simulink model "chap03_25"  (R2021a)
settings: Solver=FixedStepDiscrete  StartTime=0.0  StopTime=7.5  FixedStep=0.001  RelTol=1e-3
undefined symbols (not defined in the file): DiscIntNeverNeededParam
(part 1 of 2)
settings Model: Creator=陈天兴  LastModifiedBy=陈天兴

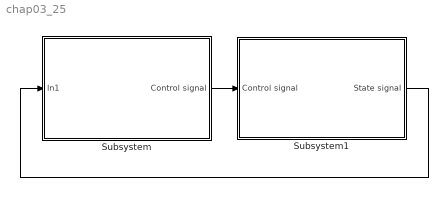
== system chap03_25 ==
  Subsystem : Subsystem
  Subsystem1 : Subsystem
  wires:
  Subsystem1/1(State signal) -> Subsystem/1(In1)
  Subsystem/1(Control signal) -> Subsystem1/1(Control signal)

== system chap03_25/Subsystem ==
  In1 : Inport
  Bus Creator : BusCreator  Inputs=6
  Bus Creator2 : BusCreator  Inputs=1
  Subsystem : Subsystem
  Subsystem1 : Subsystem
  Subsystem2 : Subsystem
  Subsystem3 : Subsystem
  Subsystem4 : Subsystem
  Subsystem5 : Subsystem
  Control signal : Outport
  wires:
  Bus Creator2/1 -> Subsystem4/1(In19), Subsystem1/1(In19), Subsystem3/1(In19), Subsystem/1(In19), Subsystem2/1(In19), Subsystem5/1(In19)
  Subsystem5/1(u3) -> Bus Creator/3
  Subsystem3/1(u4) -> Bus Creator/4
  Subsystem1/1(u5) -> Bus Creator/5
  Subsystem/1(u1) -> Bus Creator/1
  Subsystem2/1(u2) -> Bus Creator/2
  Subsystem4/1(u6) -> Bus Creator/6
  Bus Creator/1 -> Control signal/1
  In1/1 -> Bus Creator2/1  "state(t)"

== system chap03_25/Subsystem1 ==
  Control signal : Inport
  Bus Creator : BusCreator  Inputs=6
  Bus Selector : BusSelector  OutputSignals=node1.ux,node1.uy,node1.uz
  Bus Selector1 : BusSelector  OutputSignals=node2.ux,node2.uy,node2.uz
  Bus Selector2 : BusSelector  OutputSignals=node3.ux,node3.uy,node3.uz
  Bus Selector3 : BusSelector  OutputSignals=node4.ux,node4.uy,node4.uz
  Bus Selector4 : BusSelector  OutputSignals=node5.ux,node5.uy,node5.uz
  Bus Selector5 : BusSelector  OutputSignals=node6.ux,node6.uy,node6.uz
  Subsystem : Subsystem
  Subsystem1 : Subsystem
  Subsystem2 : Subsystem
  Subsystem3 : Subsystem
  Subsystem4 : Subsystem
  Subsystem5 : Subsystem
  State signal : Outport
  wires:
  Bus Creator/1 -> State signal/1
  Subsystem/1(node1) -> Bus Creator/1
  Subsystem1/1(node2) -> Bus Creator/2
  Subsystem2/1(node3) -> Bus Creator/3
  Subsystem3/1(node4) -> Bus Creator/4
  Subsystem4/1(node5) -> Bus Creator/5
  Subsystem5/1(node6) -> Bus Creator/6
  Control signal/1 -> Bus Selector2/1, Bus Selector1/1, Bus Selector/1, Bus Selector5/1, Bus Selector4/1, Bus Selector3/1
  Bus Selector/1 -> Subsystem/1(ut1x)  "<ux>"
  Bus Selector/2 -> Subsystem/2(ut1y)  "<uy>"
  Bus Selector/3 -> Subsystem/3(ut1z)  "<uz>"
  Bus Selector1/1 -> Subsystem1/1(ut2x)  "<ux>"
  Bus Selector1/2 -> Subsystem1/2(ut2y)  "<uy>"
  Bus Selector1/3 -> Subsystem1/3(ut2z)  "<uz>"
  Bus Selector2/1 -> Subsystem2/1(ut3x)  "<ux>"
  Bus Selector2/2 -> Subsystem2/2(ut3y)  "<uy>"
  Bus Selector2/3 -> Subsystem2/3(ut3z)  "<uz>"
  Bus Selector3/1 -> Subsystem3/1(ut4x)  "<ux>"
  Bus Selector3/2 -> Subsystem3/2(ut4y)  "<uy>"
  Bus Selector3/3 -> Subsystem3/3(ut4z)  "<uz>"
  Bus Selector4/1 -> Subsystem4/1(ut5x)  "<ux>"
  Bus Selector4/2 -> Subsystem4/2(ut5y)  "<uy>"
  Bus Selector4/3 -> Subsystem4/3(ut5z)  "<uz>"
  Bus Selector5/1 -> Subsystem5/1(ut6x)  "<ux>"
  Bus Selector5/2 -> Subsystem5/2(ut6y)  "<uy>"
  Bus Selector5/3 -> Subsystem5/3(ut6z)  "<uz>"

== system chap03_25/Subsystem/Subsystem ==
  In19 : Inport
  Bus Creator : BusCreator  Inputs=3
  Bus Selector : BusSelector  OutputSignals=state(t).node1.xx,state(t).node2.xx,state(t).node3.xx,state(t).node6.xx,state(t).node1.vx,state(t).node2.vx,state(t).node3.vx,state(t).node6.vx
  Bus Selector1 : BusSelector  OutputSignals=state(t).node1.xy,state(t).node2.xy,state(t).node3.xy,state(t).node6.xy,state(t).node1.vy,state(t).node2.vy,state(t).node3.vy,state(t).node6.vy
  Bus Selector2 : BusSelector  OutputSignals=state(t).node1.xz,state(t).node2.xz,state(t).node3.xz,state(t).node6.xz,state(t).node1.vz,state(t).node2.vz,state(t).node3.vz,state(t).node6.vz
  Subsystem1 : Subsystem
  Subsystem2 : Subsystem
  Subsystem6 : Subsystem
  u1 : Outport
  wires:
  Subsystem2/1(utx) -> Bus Creator/3  "uz"
  Subsystem6/1(utx) -> Bus Creator/1  "ux"
  Subsystem1/1(utx) -> Bus Creator/2  "uy"
  Bus Creator/1 -> u1/1  "node1"
  In19/1 -> Bus Selector2/1, Bus Selector1/1, Bus Selector/1
  Bus Selector/1 -> Subsystem6/1(xx1)  "<xx>"
  Bus Selector/2 -> Subsystem6/2(xx2)  "<xx>"
  Bus Selector/3 -> Subsystem6/3(xx3)  "<xx>"
  Bus Selector/4 -> Subsystem6/4(xx6)  "<xx>"
  Bus Selector/5 -> Subsystem6/5(vx1)  "<vx>"
  Bus Selector/6 -> Subsystem6/6(vx2)  "<vx>"
  Bus Selector/7 -> Subsystem6/7(vx3)  "<vx>"
  Bus Selector/8 -> Subsystem6/8(vx6)  "<vx>"
  Bus Selector1/1 -> Subsystem1/1(xy1)  "<xy>"
  Bus Selector1/2 -> Subsystem1/2(xy2)  "<xy>"
  Bus Selector1/3 -> Subsystem1/3(xy3)  "<xy>"
  Bus Selector1/4 -> Subsystem1/4(xy6)  "<xy>"
  Bus Selector1/5 -> Subsystem1/5(vy1)  "<vy>"
  Bus Selector1/6 -> Subsystem1/6(vy2)  "<vy>"
  Bus Selector1/7 -> Subsystem1/7(vy3)  "<vy>"
  Bus Selector1/8 -> Subsystem1/8(vy6)  "<vy>"
  Bus Selector2/1 -> Subsystem2/1(xz1)  "<xz>"
  Bus Selector2/2 -> Subsystem2/2(xx2)  "<xz>"
  Bus Selector2/3 -> Subsystem2/3(xz3)  "<xz>"
  Bus Selector2/4 -> Subsystem2/4(xz6)  "<xz>"
  Bus Selector2/5 -> Subsystem2/5(vz1)  "<vz>"
  Bus Selector2/6 -> Subsystem2/6(vz2)  "<vz>"
  Bus Selector2/7 -> Subsystem2/7(vz3)  "<vz>"
  Bus Selector2/8 -> Subsystem2/8(vz6)  "<vz>"

== system chap03_25/Subsystem/Subsystem1 ==
  In19 : Inport
  Bus Creator : BusCreator  Inputs=3
  Bus Selector : BusSelector  OutputSignals=state(t).node5.xx,state(t).node3.xx,state(t).node4.xx,state(t).node5.vx,state(t).node3.vx,state(t).node4.vx
  Bus Selector1 : BusSelector  OutputSignals=state(t).node5.xy,state(t).node3.xy,state(t).node4.xy,state(t).node5.vy,state(t).node3.vy,state(t).node4.vy
  Bus Selector2 : BusSelector  OutputSignals=state(t).node5.xz,state(t).node3.xz,state(t).node4.xz,state(t).node5.vz,state(t).node3.vz,state(t).node4.vz
  Subsystem2 : Subsystem
  Subsystem5 : Subsystem
  Subsystem6 : Subsystem
  u5 : Outport
  wires:
  Bus Creator/1 -> u5/1  "node5"
  Subsystem5/1(uty) -> Bus Creator/2  "uy"
  Subsystem6/1(utx) -> Bus Creator/1  "ux"
  Subsystem2/1(utz) -> Bus Creator/3  "uz"
  Bus Selector1/3 -> Subsystem5/3(xy4)  "<xy>"
  Bus Selector1/2 -> Subsystem5/2(xy3)  "<xy>"
  Bus Selector1/1 -> Subsystem5/1(xy5)  "<xy>"
  Bus Selector2/2 -> Subsystem2/2(xz3)  "<xz>"
  Bus Selector2/6 -> Subsystem2/6(vz4)  "<vz>"
  Bus Selector2/5 -> Subsystem2/5(vz3)  "<vz>"
  Bus Selector/4 -> Subsystem6/4(vx5)  "<vx>"
  Bus Selector1/6 -> Subsystem5/6(vy4)  "<vy>"
  Bus Selector1/4 -> Subsystem5/4(vy5)  "<vy>"
  In19/1 -> Bus Selector2/1, Bus Selector1/1, Bus Selector/1
  Bus Selector/1 -> Subsystem6/1(xx5)  "<xx>"
  Bus Selector/2 -> Subsystem6/2(xx3)  "<xx>"
  Bus Selector1/5 -> Subsystem5/5(vy3)  "<vy>"
  Bus Selector/6 -> Subsystem6/6(vx4)  "<vx>"
  Bus Selector/5 -> Subsystem6/5(vx3)  "<vx>"
  Bus Selector/3 -> Subsystem6/3(xx4)  "<xx>"
  Bus Selector2/1 -> Subsystem2/1(xz5)  "<xz>"
  Bus Selector2/3 -> Subsystem2/3(xz4)  "<xz>"
  Bus Selector2/4 -> Subsystem2/4(vz5)  "<vz>"

== system chap03_25/Subsystem/Subsystem2 ==
  In19 : Inport
  Bus Creator : BusCreator  Inputs=3
  Bus Selector : BusSelector  OutputSignals=state(t).node2.xx,state(t).node1.xx,state(t).node4.xx,state(t).node6.xx,state(t).node2.vx,state(t).node1.vx,state(t).node4.vx,state(t).node6.vx
  Bus Selector1 : BusSelector  OutputSignals=state(t).node2.xy,state(t).node1.xy,state(t).node4.xy,state(t).node6.xy,state(t).node2.vy,state(t).node1.vy,state(t).node4.vy,state(t).node6.vy
  Bus Selector2 : BusSelector  OutputSignals=state(t).node2.xz,state(t).node1.xz,state(t).node4.xz,state(t).node6.xz,state(t).node2.vz,state(t).node1.vz,state(t).node4.vz,state(t).node6.vz
  Subsystem1 : Subsystem
  Subsystem2 : Subsystem
  Subsystem6 : Subsystem
  u2 : Outport
  wires:
  Bus Creator/1 -> u2/1  "node2"
  Subsystem1/1(uty) -> Bus Creator/2  "uy"
  Subsystem6/1(utx) -> Bus Creator/1  "ux"
  Subsystem2/1(utz) -> Bus Creator/3  "uz"
  Bus Selector2/1 -> Subsystem2/1(xz2)  "<xz>"
  In19/1 -> Bus Selector2/1, Bus Selector1/1, Bus Selector/1
  Bus Selector/3 -> Subsystem6/3(xx4)  "<xx>"
  Bus Selector/5 -> Subsystem6/5(vx2)  "<vx>"
  Bus Selector/1 -> Subsystem6/1(xx2)  "<xx>"
  Bus Selector/7 -> Subsystem6/7(vx4)  "<vx>"
  Bus Selector1/2 -> Subsystem1/2(xy1)  "<xy>"
  Bus Selector2/4 -> Subsystem2/4(xz6)  "<xz>"
  Bus Selector2/6 -> Subsystem2/6(vz1)  "<vz>"
  Bus Selector1/1 -> Subsystem1/1(xy2)  "<xy>"
  Bus Selector2/7 -> Subsystem2/7(vz4)  "<vz>"
  Bus Selector2/5 -> Subsystem2/5(vz2)  "<vz>"
  Bus Selector1/6 -> Subsystem1/6(vy1)  "<vy>"
  Bus Selector/2 -> Subsystem6/2(xx1)  "<xx>"
  Bus Selector1/8 -> Subsystem1/8(vy6)  "<vy>"
  Bus Selector2/8 -> Subsystem2/8(vz6)  "<vz>"
  Bus Selector1/7 -> Subsystem1/7(vy4)  "<vy>"
  Bus Selector2/2 -> Subsystem2/2(xz1)  "<xz>"
  Bus Selector/8 -> Subsystem6/8(vx6)  "<vx>"
  Bus Selector1/3 -> Subsystem1/3(xy4)  "<xy>"
  Bus Selector/6 -> Subsystem6/6(vx1)  "<vx>"
  Bus Selector1/4 -> Subsystem1/4(xy6)  "<xy>"
  Bus Selector1/5 -> Subsystem1/5(vy2)  "<vy>"
  Bus Selector2/3 -> Subsystem2/3(xz4)  "<xz>"
  Bus Selector/4 -> Subsystem6/4(xx6)  "<xx>"

== system chap03_25/Subsystem/Subsystem3 ==
  In19 : Inport
  Bus Creator : BusCreator  Inputs=3
  Bus Selector : BusSelector  OutputSignals=state(t).node4.xx,state(t).node2.xx,state(t).node3.xx,state(t).node5.xx,state(t).node4.vx,state(t).node2.vx,state(t).node3.vx,state(t).node5.vx
  Bus Selector1 : BusSelector  OutputSignals=state(t).node4.xy,state(t).node2.xy,state(t).node3.xy,state(t).node5.xy,state(t).node4.vy,state(t).node2.vy,state(t).node3.vy,state(t).node5.vy
  Bus Selector2 : BusSelector  OutputSignals=state(t).node4.xz,state(t).node2.xz,state(t).node3.xz,state(t).node5.xz,state(t).node4.vz,state(t).node2.vz,state(t).node3.vz,state(t).node5.vz
  Subsystem1 : Subsystem
  Subsystem2 : Subsystem
  Subsystem6 : Subsystem
  u4 : Outport
  wires:
  Bus Creator/1 -> u4/1  "node4"
  Subsystem1/1(utx) -> Bus Creator/2  "uy"
  Subsystem6/1(utx) -> Bus Creator/1  "ux"
  Subsystem2/1(utx) -> Bus Creator/3  "uz"
  Bus Selector/2 -> Subsystem6/2(xx2)  "<xx>"
  Bus Selector1/7 -> Subsystem1/7(vy3)  "<vy>"
  Bus Selector1/4 -> Subsystem1/4(xy5)  "<xy>"
  Bus Selector2/3 -> Subsystem2/3(xz3)  "<xz>"
  Bus Selector/8 -> Subsystem6/8(vx5)  "<vx>"
  Bus Selector2/2 -> Subsystem2/2(xx2)  "<xz>"
  Bus Selector2/4 -> Subsystem2/4(xz5)  "<xz>"
  Bus Selector1/5 -> Subsystem1/5(vy4)  "<vy>"
  Bus Selector1/2 -> Subsystem1/2(xy2)  "<xy>"
  Bus Selector2/7 -> Subsystem2/7(vz3)  "<vz>"
  Bus Selector2/5 -> Subsystem2/5(vz4)  "<vz>"
  Bus Selector1/6 -> Subsystem1/6(vy2)  "<vy>"
  Bus Selector2/8 -> Subsystem2/8(vz5)  "<vz>"
  Bus Selector2/6 -> Subsystem2/6(vz2)  "<vz>"
  Bus Selector1/3 -> Subsystem1/3(xy3)  "<xy>"
  Bus Selector2/1 -> Subsystem2/1(xz4)  "<xz>"
  Bus Selector/5 -> Subsystem6/5(vx4)  "<vx>"
  Bus Selector/1 -> Subsystem6/1(xx4)  "<xx>"
  Bus Selector/3 -> Subsystem6/3(xx3)  "<xx>"
  In19/1 -> Bus Selector2/1, Bus Selector1/1, Bus Selector/1
  Bus Selector1/8 -> Subsystem1/8(vy5)  "<vy>"
  Bus Selector1/1 -> Subsystem1/1(xy4)  "<xy>"
  Bus Selector/7 -> Subsystem6/7(vx3)  "<vx>"
  Bus Selector/6 -> Subsystem6/6(vx2)  "<vx>"
  Bus Selector/4 -> Subsystem6/4(xx5)  "<xx>"

== system chap03_25/Subsystem/Subsystem4 ==
  In19 : Inport
  Bus Creator : BusCreator  Inputs=3
  Bus Selector : BusSelector  OutputSignals=state(t).node6.xx,state(t).node1.xx,state(t).node2.xx,state(t).node6.vx,state(t).node1.vx,state(t).node2.vx
  Bus Selector1 : BusSelector  OutputSignals=state(t).node6.xy,state(t).node1.xy,state(t).node2.xy,state(t).node6.vy,state(t).node1.vy,state(t).node2.vy
  Bus Selector2 : BusSelector  OutputSignals=state(t).node6.xz,state(t).node1.xz,state(t).node2.xz,state(t).node6.vz,state(t).node1.vz,state(t).node2.vz
  Subsystem1 : Subsystem
  Subsystem2 : Subsystem
  Subsystem6 : Subsystem
  u6 : Outport
  wires:
  Subsystem2/1(utz) -> Bus Creator/3  "uz"
  Subsystem6/1(utx) -> Bus Creator/1  "ux"
  Subsystem1/1(uty) -> Bus Creator/2  "uy"
  Bus Creator/1 -> u6/1  "node6"
  Bus Selector/1 -> Subsystem6/1(xx6)  "<xx>"
  Bus Selector/2 -> Subsystem6/2(xx1)  "<xx>"
  In19/1 -> Bus Selector2/1, Bus Selector1/1, Bus Selector/1
  Bus Selector2/3 -> Subsystem2/3(xz2)  "<xz>"
  Bus Selector/3 -> Subsystem6/3(xx2)  "<xx>"
  Bus Selector1/1 -> Subsystem1/1(xy6)  "<xy>"
  Bus Selector/4 -> Subsystem6/4(vx6)  "<vx>"
  Bus Selector1/2 -> Subsystem1/2(xy1)  "<xy>"
  Bus Selector/5 -> Subsystem6/5(vx1)  "<vx>"
  Bus Selector1/3 -> Subsystem1/3(xy2)  "<xy>"
  Bus Selector2/5 -> Subsystem2/5(vz1)  "<vz>"
  Bus Selector1/4 -> Subsystem1/4(vy6)  "<vy>"
  Bus Selector1/5 -> Subsystem1/5(vy1)  "<vy>"
  Bus Selector1/6 -> Subsystem1/6(vy2)  "<vy>"
  Bus Selector2/4 -> Subsystem2/4(vz6)  "<vz>"
  Bus Selector/6 -> Subsystem6/6(vx2)  "<vx>"
  Bus Selector2/2 -> Subsystem2/2(xz1)  "<xz>"
  Bus Selector2/1 -> Subsystem2/1(xz6)  "<xz>"
  Bus Selector2/6 -> Subsystem2/6(vz2)  "<vz>"

== system chap03_25/Subsystem/Subsystem5 ==
  In19 : Inport
  Bus Creator : BusCreator  Inputs=3
  Bus Selector : BusSelector  OutputSignals=state(t).node3.xx,state(t).node1.xx,state(t).node4.xx,state(t).node5.xx,state(t).node3.vx,state(t).node1.vx,state(t).node4.vx,state(t).node5.vx
  Bus Selector1 : BusSelector  OutputSignals=state(t).node3.xy,state(t).node1.xy,state(t).node4.xy,state(t).node5.xy,state(t).node3.vy,state(t).node1.vy,state(t).node4.vy,state(t).node5.vy
  Bus Selector2 : BusSelector  OutputSignals=state(t).node3.xz,state(t).node1.xz,state(t).node4.xz,state(t).node5.xz,state(t).node3.vz,state(t).node1.vz,state(t).node4.vz,state(t).node5.vz
  Subsystem1 : Subsystem
  Subsystem2 : Subsystem
  Subsystem6 : Subsystem
  u3 : Outport
  wires:
  Subsystem2/1(utz) -> Bus Creator/3  "uz"
  Subsystem6/1(utx) -> Bus Creator/1  "ux"
  Subsystem1/1(uty) -> Bus Creator/2  "uy"
  Bus Creator/1 -> u3/1  "node3"
  Bus Selector/7 -> Subsystem6/7(vx4)  "<vx>"
  In19/1 -> Bus Selector2/1, Bus Selector1/1, Bus Selector/1
  Bus Selector2/6 -> Subsystem2/6(vz1)  "<vz>"
  Bus Selector/8 -> Subsystem6/8(vx5)  "<vx>"
  Bus Selector1/1 -> Subsystem1/1(xy3)  "<xy>"
  Bus Selector/2 -> Subsystem6/2(xx1)  "<xx>"
  Bus Selector2/3 -> Subsystem2/3(xz4)  "<xz>"
  Bus Selector2/2 -> Subsystem2/2(xz1)  "<xz>"
  Bus Selector/5 -> Subsystem6/5(vx3)  "<vx>"
  Bus Selector/1 -> Subsystem6/1(xx3)  "<xx>"
  Bus Selector1/7 -> Subsystem1/7(vy4)  "<vy>"
  Bus Selector/3 -> Subsystem6/3(xx4)  "<xx>"
  Bus Selector/6 -> Subsystem6/6(vx1)  "<vx>"
  Bus Selector1/2 -> Subsystem1/2(xy1)  "<xy>"
  Bus Selector1/5 -> Subsystem1/5(vy3)  "<vy>"
  Bus Selector1/8 -> Subsystem1/8(vy5)  "<vy>"
  Bus Selector2/1 -> Subsystem2/1(xz3)  "<xz>"
  Bus Selector1/4 -> Subsystem1/4(xy5)  "<xy>"
  Bus Selector1/3 -> Subsystem1/3(xy4)  "<xy>"
  Bus Selector/4 -> Subsystem6/4(xx5)  "<xx>"
  Bus Selector2/5 -> Subsystem2/5(vz3)  "<vz>"
  Bus Selector2/7 -> Subsystem2/7(vz4)  "<vz>"
  Bus Selector1/6 -> Subsystem1/6(vy1)  "<vy>"
  Bus Selector2/8 -> Subsystem2/8(vz5)  "<vz>"
  Bus Selector2/4 -> Subsystem2/4(xz5)  "<xz>"

== system chap03_25/Subsystem1/Subsystem ==
  ut1x : Inport
  ut1y : Inport  Port=2
  ut1z : Inport  Port=3
  Bus Creator1 : BusCreator  Inputs=6
  Discrete-Time Integrator : DiscreteIntegrator  SampleTime=-1  ICPrevOutput=DiscIntNeverNeededParam  ICPrevScaledInput=DiscIntNeverNeededParam
  Discrete-Time Integrator14 : DiscreteIntegrator  InitialCondition=-2.7  SampleTime=-1  ICPrevOutput=DiscIntNeverNeededParam  ICPrevScaledInput=DiscIntNeverNeededParam
  Discrete-Time Integrator15 : DiscreteIntegrator  InitialCondition=2.5  SampleTime=-1  ICPrevOutput=DiscIntNeverNeededParam  ICPrevScaledInput=DiscIntNeverNeededParam
  Discrete-Time Integrator16 : DiscreteIntegrator  InitialCondition=0.17  SampleTime=-1  ICPrevOutput=DiscIntNeverNeededParam  ICPrevScaledInput=DiscIntNeverNeededParam
  Discrete-Time Integrator17 : DiscreteIntegrator  SampleTime=-1  ICPrevOutput=DiscIntNeverNeededParam  ICPrevScaledInput=DiscIntNeverNeededParam
  Discrete-Time Integrator5 : DiscreteIntegrator  InitialCondition=-2.9  SampleTime=-1  ICPrevOutput=DiscIntNeverNeededParam  ICPrevScaledInput=DiscIntNeverNeededParam
  node1 : Outport
  wires:
  ut1y/1 -> Discrete-Time Integrator17/1
  ut1z/1 -> Discrete-Time Integrator/1
  Discrete-Time Integrator17/1 -> Discrete-Time Integrator15/1, Bus Creator1/5  "vy"
  Discrete-Time Integrator/1 -> Discrete-Time Integrator5/1, Bus Creator1/6  "vz"
  ut1x/1 -> Discrete-Time Integrator16/1
  Discrete-Time Integrator16/1 -> Bus Creator1/4, Discrete-Time Integrator14/1  "vx"
  Bus Creator1/1 -> node1/1  "node1"
  Discrete-Time Integrator5/1 -> Bus Creator1/3  "xz"
  Discrete-Time Integrator15/1 -> Bus Creator1/2  "xy"
  Discrete-Time Integrator14/1 -> Bus Creator1/1  "xx"

== system chap03_25/Subsystem1/Subsystem1 ==
  ut2x : Inport
  ut2y : Inport  Port=2
  ut2z : Inport  Port=3
  Bus Creator1 : BusCreator  Inputs=6
  Discrete-Time Integrator1 : DiscreteIntegrator  SampleTime=-1  ICPrevOutput=DiscIntNeverNeededParam  ICPrevScaledInput=DiscIntNeverNeededParam
  Discrete-Time Integrator14 : DiscreteIntegrator  InitialCondition=-1.7  SampleTime=-1  ICPrevOutput=DiscIntNeverNeededParam  ICPrevScaledInput=DiscIntNeverNeededParam
  Discrete-Time Integrator15 : DiscreteIntegrator  InitialCondition=-1.4  SampleTime=-1  ICPrevOutput=DiscIntNeverNeededParam  ICPrevScaledInput=DiscIntNeverNeededParam
  Discrete-Time Integrator2 : DiscreteIntegrator  SampleTime=-1  ICPrevOutput=DiscIntNeverNeededParam  ICPrevScaledInput=DiscIntNeverNeededParam
  Discrete-Time Integrator3 : DiscreteIntegrator  InitialCondition=0.13  SampleTime=-1  ICPrevOutput=DiscIntNeverNeededParam  ICPrevScaledInput=DiscIntNeverNeededParam
  Discrete-Time Integrator5 : DiscreteIntegrator  InitialCondition=-1.5  SampleTime=-1  ICPrevOutput=DiscIntNeverNeededParam  ICPrevScaledInput=DiscIntNeverNeededParam
  node2 : Outport
  wires:
  Discrete-Time Integrator14/1 -> Bus Creator1/1  "xx"
  Discrete-Time Integrator15/1 -> Bus Creator1/2  "xy"
  Discrete-Time Integrator5/1 -> Bus Creator1/3  "xz"
  Bus Creator1/1 -> node2/1  "node2"
  Discrete-Time Integrator2/1 -> Discrete-Time Integrator14/1, Bus Creator1/4  "vx"
  ut2x/1 -> Discrete-Time Integrator2/1
  Discrete-Time Integrator1/1 -> Bus Creator1/6, Discrete-Time Integrator5/1  "vz"
  Discrete-Time Integrator3/1 -> Bus Creator1/5, Discrete-Time Integrator15/1  "vy"
  ut2z/1 -> Discrete-Time Integrator1/1
  ut2y/1 -> Discrete-Time Integrator3/1

== system chap03_25/Subsystem1/Subsystem2 ==
  ut3x : Inport
  ut3y : Inport  Port=2
  ut3z : Inport  Port=3
  Bus Creator1 : BusCreator  Inputs=6
  Discrete-Time Integrator : DiscreteIntegrator  InitialCondition=0.12  SampleTime=-1  ICPrevOutput=DiscIntNeverNeededParam  ICPrevScaledInput=DiscIntNeverNeededParam
  Discrete-Time Integrator14 : DiscreteIntegrator  InitialCondition=0.6  SampleTime=-1  ICPrevOutput=DiscIntNeverNeededParam  ICPrevScaledInput=DiscIntNeverNeededParam
  Discrete-Time Integrator15 : DiscreteIntegrator  InitialCondition=-0.7  SampleTime=-1  ICPrevOutput=DiscIntNeverNeededParam  ICPrevScaledInput=DiscIntNeverNeededParam
  Discrete-Time Integrator16 : DiscreteIntegrator  SampleTime=-1  ICPrevOutput=DiscIntNeverNeededParam  ICPrevScaledInput=DiscIntNeverNeededParam
  Discrete-Time Integrator17 : DiscreteIntegrator  SampleTime=-1  ICPrevOutput=DiscIntNeverNeededParam  ICPrevScaledInput=DiscIntNeverNeededParam
  Discrete-Time Integrator5 : DiscreteIntegrator  InitialCondition=0.5  SampleTime=-1  ICPrevOutput=DiscIntNeverNeededParam  ICPrevScaledInput=DiscIntNeverNeededParam
  node3 : Outport
  wires:
  ut3y/1 -> Discrete-Time Integrator17/1
  ut3z/1 -> Discrete-Time Integrator/1
  Discrete-Time Integrator17/1 -> Discrete-Time Integrator15/1, Bus Creator1/5  "vy"
  Discrete-Time Integrator/1 -> Discrete-Time Integrator5/1, Bus Creator1/6  "vz"
  ut3x/1 -> Discrete-Time Integrator16/1
  Discrete-Time Integrator16/1 -> Bus Creator1/4, Discrete-Time Integrator14/1  "vx"
  Bus Creator1/1 -> node3/1  "node3"
  Discrete-Time Integrator5/1 -> Bus Creator1/3  "xz"
  Discrete-Time Integrator15/1 -> Bus Creator1/2  "xy"
  Discrete-Time Integrator14/1 -> Bus Creator1/1  "xx"

== system chap03_25/Subsystem1/Subsystem3 ==
  ut4x : Inport
  ut4y : Inport  Port=2
  ut4z : Inport  Port=3
  Bus Creator1 : BusCreator  Inputs=6
  Discrete-Time Integrator : DiscreteIntegrator  InitialCondition=-0.15  SampleTime=-1  ICPrevOutput=DiscIntNeverNeededParam  ICPrevScaledInput=DiscIntNeverNeededParam
  Discrete-Time Integrator14 : DiscreteIntegrator  InitialCondition=-0.7  SampleTime=-1  ICPrevOutput=DiscIntNeverNeededParam  ICPrevScaledInput=DiscIntNeverNeededParam
  Discrete-Time Integrator15 : DiscreteIntegrator  InitialCondition=0.9  SampleTime=-1  ICPrevOutput=DiscIntNeverNeededParam  ICPrevScaledInput=DiscIntNeverNeededParam
  Discrete-Time Integrator16 : DiscreteIntegrator  SampleTime=-1  ICPrevOutput=DiscIntNeverNeededParam  ICPrevScaledInput=DiscIntNeverNeededParam
  Discrete-Time Integrator17 : DiscreteIntegrator  SampleTime=-1  ICPrevOutput=DiscIntNeverNeededParam  ICPrevScaledInput=DiscIntNeverNeededParam
  Discrete-Time Integrator5 : DiscreteIntegrator  InitialCondition=-0.8  SampleTime=-1  ICPrevOutput=DiscIntNeverNeededParam  ICPrevScaledInput=DiscIntNeverNeededParam
  node4 : Outport
  wires:
  Discrete-Time Integrator14/1 -> Bus Creator1/1  "xx"
  Discrete-Time Integrator15/1 -> Bus Creator1/2  "xy"
  Discrete-Time Integrator5/1 -> Bus Creator1/3  "xz"
  Bus Creator1/1 -> node4/1  "node4"
  Discrete-Time Integrator16/1 -> Discrete-Time Integrator14/1, Bus Creator1/4  "vx"
  ut4x/1 -> Discrete-Time Integrator16/1
  Discrete-Time Integrator/1 -> Bus Creator1/6, Discrete-Time Integrator5/1  "vz"
  Discrete-Time Integrator17/1 -> Bus Creator1/5, Discrete-Time Integrator15/1  "vy"
  ut4z/1 -> Discrete-Time Integrator/1
  ut4y/1 -> Discrete-Time Integrator17/1

== system chap03_25/Subsystem1/Subsystem4 ==
  ut5x : Inport
  ut5y : Inport  Port=2
  ut5z : Inport  Port=3
  Bus Creator1 : BusCreator  Inputs=6
  Discrete-Time Integrator : DiscreteIntegrator  SampleTime=-1  ICPrevOutput=DiscIntNeverNeededParam  ICPrevScaledInput=DiscIntNeverNeededParam
  Discrete-Time Integrator14 : DiscreteIntegrator  InitialCondition=1.1  SampleTime=-1  ICPrevOutput=DiscIntNeverNeededParam  ICPrevScaledInput=DiscIntNeverNeededParam
  Discrete-Time Integrator15 : DiscreteIntegrator  InitialCondition=1.6  SampleTime=-1  ICPrevOutput=DiscIntNeverNeededParam  ICPrevScaledInput=DiscIntNeverNeededParam
  Discrete-Time Integrator16 : DiscreteIntegrator  SampleTime=-1  ICPrevOutput=DiscIntNeverNeededParam  ICPrevScaledInput=DiscIntNeverNeededParam
  Discrete-Time Integrator17 : DiscreteIntegrator  InitialCondition=-0.12  SampleTime=-1  ICPrevOutput=DiscIntNeverNeededParam  ICPrevScaledInput=DiscIntNeverNeededParam
  Discrete-Time Integrator5 : DiscreteIntegrator  InitialCondition=1.4  SampleTime=-1  ICPrevOutput=DiscIntNeverNeededParam  ICPrevScaledInput=DiscIntNeverNeededParam
  node5 : Outport
  wires:
  ut5y/1 -> Discrete-Time Integrator17/1
  ut5z/1 -> Discrete-Time Integrator/1
  Discrete-Time Integrator17/1 -> Discrete-Time Integrator15/1, Bus Creator1/5  "vy"
  Discrete-Time Integrator/1 -> Discrete-Time Integrator5/1, Bus Creator1/6  "vz"
  ut5x/1 -> Discrete-Time Integrator16/1
  Discrete-Time Integrator16/1 -> Bus Creator1/4, Discrete-Time Integrator14/1  "vx"
  Bus Creator1/1 -> node5/1  "node5"
  Discrete-Time Integrator5/1 -> Bus Creator1/3  "xz"
  Discrete-Time Integrator15/1 -> Bus Creator1/2  "xy"
  Discrete-Time Integrator14/1 -> Bus Creator1/1  "xx"

== system chap03_25/Subsystem1/Subsystem5 ==
  ut6x : Inport
  ut6y : Inport  Port=2
  ut6z : Inport  Port=3
  Bus Creator1 : BusCreator  Inputs=6
  Discrete-Time Integrator : DiscreteIntegrator  SampleTime=-1  ICPrevOutput=DiscIntNeverNeededParam  ICPrevScaledInput=DiscIntNeverNeededParam
  Discrete-Time Integrator14 : DiscreteIntegrator  InitialCondition=2.7  SampleTime=-1  ICPrevOutput=DiscIntNeverNeededParam  ICPrevScaledInput=DiscIntNeverNeededParam
  Discrete-Time Integrator15 : DiscreteIntegrator  InitialCondition=-2.8  SampleTime=-1  ICPrevOutput=DiscIntNeverNeededParam  ICPrevScaledInput=DiscIntNeverNeededParam
  Discrete-Time Integrator16 : DiscreteIntegrator  InitialCondition=-0.18  SampleTime=-1  ICPrevOutput=DiscIntNeverNeededParam  ICPrevScaledInput=DiscIntNeverNeededParam
  Discrete-Time Integrator17 : DiscreteIntegrator  SampleTime=-1  ICPrevOutput=DiscIntNeverNeededParam  ICPrevScaledInput=DiscIntNeverNeededParam
  Discrete-Time Integrator5 : DiscreteIntegrator  InitialCondition=2.5  SampleTime=-1  ICPrevOutput=DiscIntNeverNeededParam  ICPrevScaledInput=DiscIntNeverNeededParam
  node6 : Outport
  wires:
  Discrete-Time Integrator14/1 -> Bus Creator1/1  "xx"
  Discrete-Time Integrator15/1 -> Bus Creator1/2  "xy"
  Discrete-Time Integrator5/1 -> Bus Creator1/3  "xz"
  Bus Creator1/1 -> node6/1  "node6"
  Discrete-Time Integrator16/1 -> Discrete-Time Integrator14/1, Bus Creator1/4  "vx"
  ut6x/1 -> Discrete-Time Integrator16/1
  Discrete-Time Integrator/1 -> Bus Creator1/6, Discrete-Time Integrator5/1  "vz"
  Discrete-Time Integrator17/1 -> Bus Creator1/5, Discrete-Time Integrator15/1  "vy"
  ut6z/1 -> Discrete-Time Integrator/1
  ut6y/1 -> Discrete-Time Integrator17/1

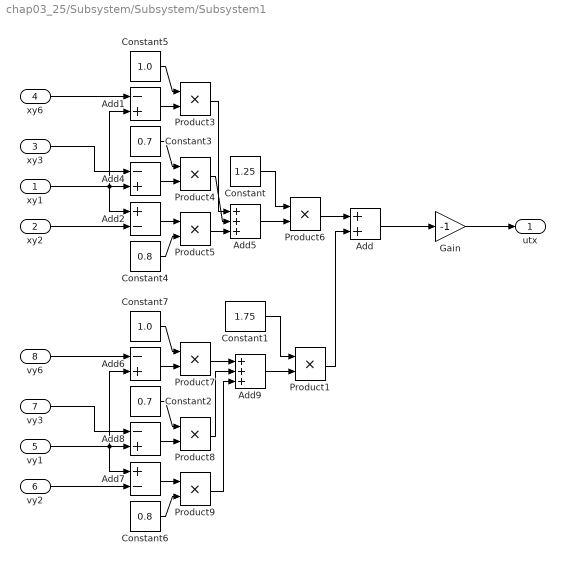
== system chap03_25/Subsystem/Subsystem/Subsystem1 ==
  xy1 : Inport
  xy2 : Inport  Port=2
  xy3 : Inport  Port=3
  xy6 : Inport  Port=4
  vy1 : Inport  Port=5
  vy2 : Inport  Port=6
  vy3 : Inport  Port=7
  vy6 : Inport  Port=8
  Add : Sum
  Add{1,4,6,8} (4 alike) : Sum  Inputs=-+
  Add2 : Sum  Inputs=+-
  Add5 : Sum  Inputs=+++
  Add7 : Sum  Inputs=+-
  Add9 : Sum  Inputs=+++
  Constant : Constant  Value=1.25
  Constant1 : Constant  Value=1.75
  Constant2 : Constant  Value=0.7
  Constant3 : Constant  Value=0.7
  Constant4 : Constant  Value=0.8
  Constant5 : Constant  Value=1.0
  Constant6 : Constant  Value=0.8
  Constant7 : Constant  Value=1.0
  Gain : Gain  Gain=-1
  Product{1,3..9} (8 alike) : Product
  utx : Outport
  wires:
  Product8/1 -> Add9/2
  Product9/1 -> Add9/3
  Constant2/1 -> Product8/1
  Add8/1 -> Product8/2
  vy1/1 -> Add6/2, Add8/2, Add7/1
  Constant6/1 -> Product9/2
  Add7/1 -> Product9/1
  vy3/1 -> Add8/1
  vy2/1 -> Add7/2
  vy6/1 -> Add6/1
  Constant7/1 -> Product7/1
  Add6/1 -> Product7/2
  Product7/1 -> Add9/1
  Product3/1 -> Add5/1
  Add1/1 -> Product3/2
  Constant5/1 -> Product3/1
  xy6/1 -> Add1/1
  xy2/1 -> Add2/2
  xy3/1 -> Add4/1
  Add5/1 -> Product6/2
  Add2/1 -> Product5/1
  Product1/1 -> Add/2
  Constant1/1 -> Product1/1
  Constant/1 -> Product6/1
  Product6/1 -> Add/1
  Constant4/1 -> Product5/2
  xy1/1 -> Add2/1, Add4/2, Add1/2
  Add4/1 -> Product4/2
  Constant3/1 -> Product4/1
  Product5/1 -> Add5/3
  Product4/1 -> Add5/2
  Add9/1 -> Product1/2
  Gain/1 -> utx/1
  Add/1 -> Gain/1

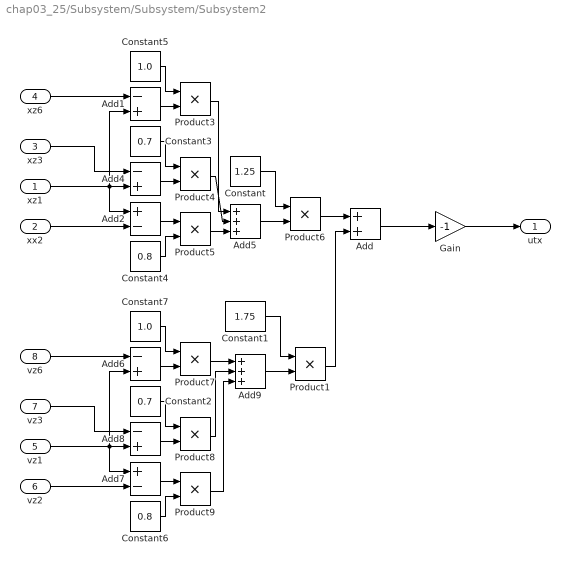
== system chap03_25/Subsystem/Subsystem/Subsystem2 ==
  xz1 : Inport
  xx2 : Inport  Port=2
  xz3 : Inport  Port=3
  xz6 : Inport  Port=4
  vz1 : Inport  Port=5
  vz2 : Inport  Port=6
  vz3 : Inport  Port=7
  vz6 : Inport  Port=8
  Add : Sum
  Add{1,4,6,8} (4 alike) : Sum  Inputs=-+
  Add2 : Sum  Inputs=+-
  Add5 : Sum  Inputs=+++
  Add7 : Sum  Inputs=+-
  Add9 : Sum  Inputs=+++
  Constant : Constant  Value=1.25
  Constant1 : Constant  Value=1.75
  Constant2 : Constant  Value=0.7
  Constant3 : Constant  Value=0.7
  Constant4 : Constant  Value=0.8
  Constant5 : Constant  Value=1.0
  Constant6 : Constant  Value=0.8
  Constant7 : Constant  Value=1.0
  Gain : Gain  Gain=-1
  Product{1,3..9} (8 alike) : Product
  utx : Outport
  wires:
  Add9/1 -> Product1/2
  Product4/1 -> Add5/2
  Product5/1 -> Add5/3
  Constant3/1 -> Product4/1
  Add4/1 -> Product4/2
  xz1/1 -> Add1/2, Add4/2, Add2/1
  Constant4/1 -> Product5/2
  Product6/1 -> Add/1
  Constant/1 -> Product6/1
  Constant1/1 -> Product1/1
  Product1/1 -> Add/2
  Add2/1 -> Product5/1
  Add5/1 -> Product6/2
  xz3/1 -> Add4/1
  xx2/1 -> Add2/2
  xz6/1 -> Add1/1
  Constant5/1 -> Product3/1
  Add1/1 -> Product3/2
  Product3/1 -> Add5/1
  Product7/1 -> Add9/1
  Add6/1 -> Product7/2
  Constant7/1 -> Product7/1
  vz6/1 -> Add6/1
  vz2/1 -> Add7/2
  vz3/1 -> Add8/1
  Add7/1 -> Product9/1
  Constant6/1 -> Product9/2
  vz1/1 -> Add7/1, Add8/2, Add6/2
  Add8/1 -> Product8/2
  Constant2/1 -> Product8/1
  Product9/1 -> Add9/3
  Product8/1 -> Add9/2
  Gain/1 -> utx/1
  Add/1 -> Gain/1

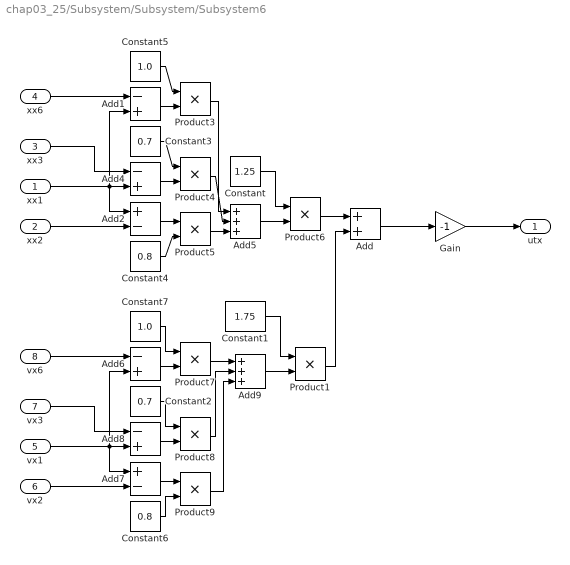
== system chap03_25/Subsystem/Subsystem/Subsystem6 ==
  xx1 : Inport
  xx2 : Inport  Port=2
  xx3 : Inport  Port=3
  xx6 : Inport  Port=4
  vx1 : Inport  Port=5
  vx2 : Inport  Port=6
  vx3 : Inport  Port=7
  vx6 : Inport  Port=8
  Add : Sum
  Add{1,4,6,8} (4 alike) : Sum  Inputs=-+
  Add2 : Sum  Inputs=+-
  Add5 : Sum  Inputs=+++
  Add7 : Sum  Inputs=+-
  Add9 : Sum  Inputs=+++
  Constant : Constant  Value=1.25
  Constant1 : Constant  Value=1.75
  Constant2 : Constant  Value=0.7
  Constant3 : Constant  Value=0.7
  Constant4 : Constant  Value=0.8
  Constant5 : Constant  Value=1.0
  Constant6 : Constant  Value=0.8
  Constant7 : Constant  Value=1.0
  Gain : Gain  Gain=-1
  Product{1,3..9} (8 alike) : Product
  utx : Outport
  wires:
  Add9/1 -> Product1/2
  Product4/1 -> Add5/2
  Product5/1 -> Add5/3
  Constant3/1 -> Product4/1
  Add4/1 -> Product4/2
  xx1/1 -> Add1/2, Add4/2, Add2/1
  Constant4/1 -> Product5/2
  Product6/1 -> Add/1
  Constant/1 -> Product6/1
  Constant1/1 -> Product1/1
  Product1/1 -> Add/2
  Add2/1 -> Product5/1
  Add5/1 -> Product6/2
  Add/1 -> Gain/1
  xx3/1 -> Add4/1
  xx2/1 -> Add2/2
  xx6/1 -> Add1/1
  Constant5/1 -> Product3/1
  Add1/1 -> Product3/2
  Product3/1 -> Add5/1
  Product7/1 -> Add9/1
  Add6/1 -> Product7/2
  Constant7/1 -> Product7/1
  vx6/1 -> Add6/1
  vx2/1 -> Add7/2
  vx3/1 -> Add8/1
  Add7/1 -> Product9/1
  Constant6/1 -> Product9/2
  vx1/1 -> Add7/1, Add8/2, Add6/2
  Add8/1 -> Product8/2
  Constant2/1 -> Product8/1
  Product9/1 -> Add9/3
  Product8/1 -> Add9/2
  Gain/1 -> utx/1

== system chap03_25/Subsystem/Subsystem1/Subsystem2 ==
  xz5 : Inport
  xz3 : Inport  Port=2
  xz4 : Inport  Port=3
  vz5 : Inport  Port=4
  vz3 : Inport  Port=5
  vz4 : Inport  Port=6
  Add : Sum
  Add10 : Sum  Inputs=-+
  Add2 : Sum  Inputs=+-
  Add4 : Sum  Inputs=-+
  Add5 : Sum
  Add8 : Sum
  Add9 : Sum  Inputs=+-
  Constant : Constant  Value=1.25
  Constant1 : Constant  Value=1.75
  Constant3 : Constant  Value=1.0
  Constant4 : Constant  Value=1.2
  Constant5 : Constant  Value=1.0
  Constant6 : Constant  Value=1.2
  Gain : Gain  Gain=-1
  Product{1,4..6,8..9} (6 alike) : Product
  utz : Outport
  wires:
  vz5/1 -> Add9/1, Add10/2
  vz4/1 -> Add10/1
  vz3/1 -> Add9/2
  xz3/1 -> Add2/2
  xz4/1 -> Add4/1
  Add5/1 -> Product6/2
  Add2/1 -> Product5/1
  Product1/1 -> Add/2
  Constant1/1 -> Product1/1
  Constant/1 -> Product6/1
  Product6/1 -> Add/1
  Constant4/1 -> Product5/2
  xz5/1 -> Add4/2, Add2/1
  Add4/1 -> Product4/2
  Constant3/1 -> Product4/1
  Product5/1 -> Add5/2
  Product4/1 -> Add5/1
  Add8/1 -> Product1/2
  Constant5/1 -> Product8/1
  Add10/1 -> Product8/2
  Constant6/1 -> Product9/2
  Add9/1 -> Product9/1
  Product8/1 -> Add8/1
  Product9/1 -> Add8/2
  Gain/1 -> utz/1
  Add/1 -> Gain/1

== system chap03_25/Subsystem/Subsystem1/Subsystem5 ==
  xy5 : Inport
  xy3 : Inport  Port=2
  xy4 : Inport  Port=3
  vy5 : Inport  Port=4
  vy3 : Inport  Port=5
  vy4 : Inport  Port=6
  Add : Sum
  Add10 : Sum  Inputs=-+
  Add2 : Sum  Inputs=+-
  Add4 : Sum  Inputs=-+
  Add5 : Sum
  Add8 : Sum
  Add9 : Sum  Inputs=+-
  Constant : Constant  Value=1.25
  Constant1 : Constant  Value=1.75
  Constant3 : Constant  Value=1.0
  Constant4 : Constant  Value=1.2
  Constant5 : Constant  Value=1.0
  Constant6 : Constant  Value=1.2
  Gain : Gain  Gain=-1
  Product{1,4..6,8..9} (6 alike) : Product
  uty : Outport
  wires:
  Product9/1 -> Add8/2
  Product8/1 -> Add8/1
  Add9/1 -> Product9/1
  Constant6/1 -> Product9/2
  Add10/1 -> Product8/2
  Constant5/1 -> Product8/1
  Add8/1 -> Product1/2
  Product4/1 -> Add5/1
  Product5/1 -> Add5/2
  Constant3/1 -> Product4/1
  Add4/1 -> Product4/2
  xy5/1 -> Add2/1, Add4/2
  Constant4/1 -> Product5/2
  Product6/1 -> Add/1
  Constant/1 -> Product6/1
  Constant1/1 -> Product1/1
  Product1/1 -> Add/2
  Add2/1 -> Product5/1
  Add5/1 -> Product6/2
  xy4/1 -> Add4/1
  xy3/1 -> Add2/2
  vy3/1 -> Add9/2
  vy4/1 -> Add10/1
  vy5/1 -> Add10/2, Add9/1
  Gain/1 -> uty/1
  Add/1 -> Gain/1

== system chap03_25/Subsystem/Subsystem1/Subsystem6 ==
  xx5 : Inport
  xx3 : Inport  Port=2
  xx4 : Inport  Port=3
  vx5 : Inport  Port=4
  vx3 : Inport  Port=5
  vx4 : Inport  Port=6
  Add : Sum
  Add10 : Sum  Inputs=-+
  Add2 : Sum  Inputs=+-
  Add4 : Sum  Inputs=-+
  Add5 : Sum
  Add8 : Sum
  Add9 : Sum  Inputs=+-
  Constant : Constant  Value=1.25
  Constant1 : Constant  Value=1.75
  Constant3 : Constant  Value=1.0
  Constant4 : Constant  Value=1.2
  Constant5 : Constant  Value=1.0
  Constant6 : Constant  Value=1.2
  Gain : Gain  Gain=-1
  Product{1,4..6,8..9} (6 alike) : Product
  utx : Outport
  wires:
  vx5/1 -> Add9/1, Add10/2
  vx4/1 -> Add10/1
  vx3/1 -> Add9/2
  xx3/1 -> Add2/2
  xx4/1 -> Add4/1
  Add5/1 -> Product6/2
  Add2/1 -> Product5/1
  Product1/1 -> Add/2
  Constant1/1 -> Product1/1
  Constant/1 -> Product6/1
  Product6/1 -> Add/1
  Constant4/1 -> Product5/2
  xx5/1 -> Add4/2, Add2/1
  Add4/1 -> Product4/2
  Constant3/1 -> Product4/1
  Product5/1 -> Add5/2
  Product4/1 -> Add5/1
  Add8/1 -> Product1/2
  Constant5/1 -> Product8/1
  Add10/1 -> Product8/2
  Constant6/1 -> Product9/2
  Add9/1 -> Product9/1
  Product8/1 -> Add8/1
  Product9/1 -> Add8/2
  Gain/1 -> utx/1
  Add/1 -> Gain/1

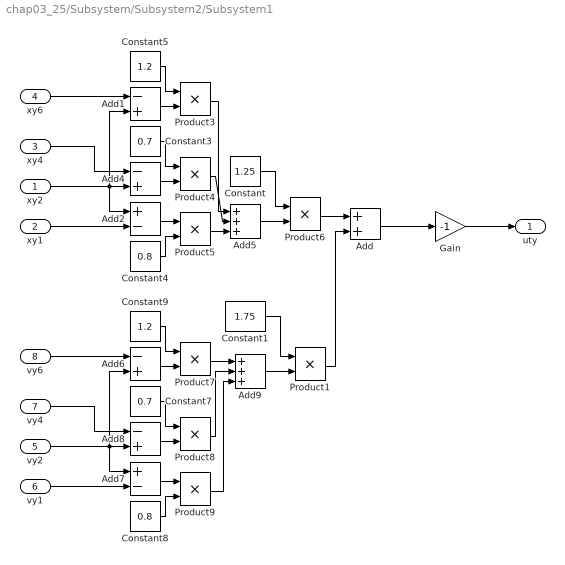
== system chap03_25/Subsystem/Subsystem2/Subsystem1 ==
  xy2 : Inport
  xy1 : Inport  Port=2
  xy4 : Inport  Port=3
  xy6 : Inport  Port=4
  vy2 : Inport  Port=5
  vy1 : Inport  Port=6
  vy4 : Inport  Port=7
  vy6 : Inport  Port=8
  Add : Sum
  Add{1,4,6,8} (4 alike) : Sum  Inputs=-+
  Add2 : Sum  Inputs=+-
  Add5 : Sum  Inputs=+++
  Add7 : Sum  Inputs=+-
  Add9 : Sum  Inputs=+++
  Constant : Constant  Value=1.25
  Constant1 : Constant  Value=1.75
  Constant3 : Constant  Value=0.7
  Constant4 : Constant  Value=0.8
  Constant5 : Constant  Value=1.2
  Constant7 : Constant  Value=0.7
  Constant8 : Constant  Value=0.8
  Constant9 : Constant  Value=1.2
  Gain : Gain  Gain=-1
  Product{1,3..9} (8 alike) : Product
  uty : Outport
  wires:
  Add9/1 -> Product1/2
  Product4/1 -> Add5/2
  Product5/1 -> Add5/3
  Constant3/1 -> Product4/1
  Add4/1 -> Product4/2
  xy2/1 -> Add1/2, Add4/2, Add2/1
  Constant4/1 -> Product5/2
  Product6/1 -> Add/1
  Constant/1 -> Product6/1
  Constant1/1 -> Product1/1
  Product1/1 -> Add/2
  Add2/1 -> Product5/1
  Add5/1 -> Product6/2
  xy4/1 -> Add4/1
  xy1/1 -> Add2/2
  xy6/1 -> Add1/1
  Constant5/1 -> Product3/1
  Add1/1 -> Product3/2
  Product3/1 -> Add5/1
  Product7/1 -> Add9/1
  Add6/1 -> Product7/2
  Constant9/1 -> Product7/1
  vy6/1 -> Add6/1
  vy1/1 -> Add7/2
  vy4/1 -> Add8/1
  Add7/1 -> Product9/1
  Constant8/1 -> Product9/2
  vy2/1 -> Add7/1, Add8/2, Add6/2
  Add8/1 -> Product8/2
  Constant7/1 -> Product8/1
  Product9/1 -> Add9/3
  Product8/1 -> Add9/2
  Gain/1 -> uty/1
  Add/1 -> Gain/1

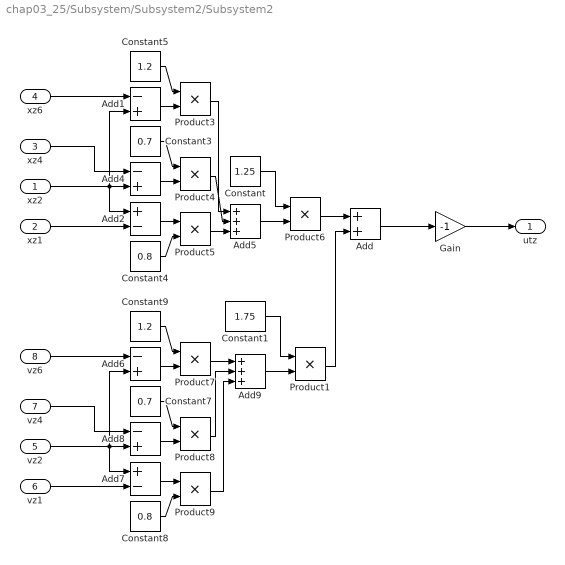
== system chap03_25/Subsystem/Subsystem2/Subsystem2 ==
  xz2 : Inport
  xz1 : Inport  Port=2
  xz4 : Inport  Port=3
  xz6 : Inport  Port=4
  vz2 : Inport  Port=5
  vz1 : Inport  Port=6
  vz4 : Inport  Port=7
  vz6 : Inport  Port=8
  Add : Sum
  Add{1,4,6,8} (4 alike) : Sum  Inputs=-+
  Add2 : Sum  Inputs=+-
  Add5 : Sum  Inputs=+++
  Add7 : Sum  Inputs=+-
  Add9 : Sum  Inputs=+++
  Constant : Constant  Value=1.25
  Constant1 : Constant  Value=1.75
  Constant3 : Constant  Value=0.7
  Constant4 : Constant  Value=0.8
  Constant5 : Constant  Value=1.2
  Constant7 : Constant  Value=0.7
  Constant8 : Constant  Value=0.8
  Constant9 : Constant  Value=1.2
  Gain : Gain  Gain=-1
  Product{1,3..9} (8 alike) : Product
  utz : Outport
  wires:
  Product8/1 -> Add9/2
  Product9/1 -> Add9/3
  Constant7/1 -> Product8/1
  Add8/1 -> Product8/2
  vz2/1 -> Add6/2, Add8/2, Add7/1
  Constant8/1 -> Product9/2
  Add7/1 -> Product9/1
  vz4/1 -> Add8/1
  vz1/1 -> Add7/2
  vz6/1 -> Add6/1
  Constant9/1 -> Product7/1
  Add6/1 -> Product7/2
  Product7/1 -> Add9/1
  Product3/1 -> Add5/1
  Add1/1 -> Product3/2
  Constant5/1 -> Product3/1
  xz6/1 -> Add1/1
  xz1/1 -> Add2/2
  xz4/1 -> Add4/1
  Add5/1 -> Product6/2
  Add2/1 -> Product5/1
  Product1/1 -> Add/2
  Constant1/1 -> Product1/1
  Constant/1 -> Product6/1
  Product6/1 -> Add/1
  Constant4/1 -> Product5/2
  xz2/1 -> Add2/1, Add4/2, Add1/2
  Add4/1 -> Product4/2
  Constant3/1 -> Product4/1
  Product5/1 -> Add5/3
  Product4/1 -> Add5/2
  Add9/1 -> Product1/2
  Gain/1 -> utz/1
  Add/1 -> Gain/1

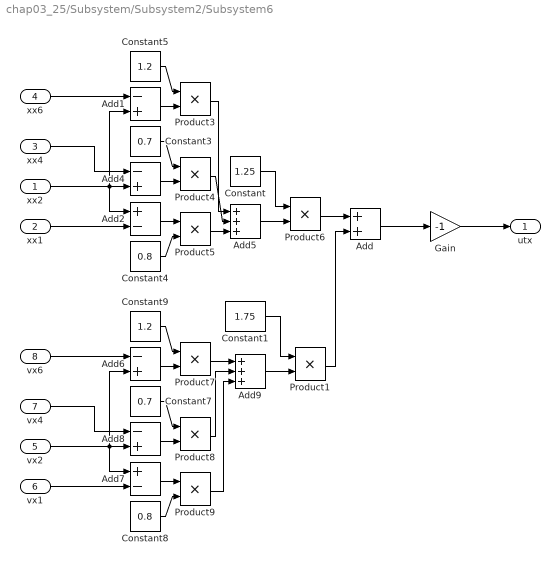
== system chap03_25/Subsystem/Subsystem2/Subsystem6 ==
  xx2 : Inport
  xx1 : Inport  Port=2
  xx4 : Inport  Port=3
  xx6 : Inport  Port=4
  vx2 : Inport  Port=5
  vx1 : Inport  Port=6
  vx4 : Inport  Port=7
  vx6 : Inport  Port=8
  Add : Sum
  Add{1,4,6,8} (4 alike) : Sum  Inputs=-+
  Add2 : Sum  Inputs=+-
  Add5 : Sum  Inputs=+++
  Add7 : Sum  Inputs=+-
  Add9 : Sum  Inputs=+++
  Constant : Constant  Value=1.25
  Constant1 : Constant  Value=1.75
  Constant3 : Constant  Value=0.7
  Constant4 : Constant  Value=0.8
  Constant5 : Constant  Value=1.2
  Constant7 : Constant  Value=0.7
  Constant8 : Constant  Value=0.8
  Constant9 : Constant  Value=1.2
  Gain : Gain  Gain=-1
  Product{1,3..9} (8 alike) : Product
  utx : Outport
  wires:
  Product8/1 -> Add9/2
  Product9/1 -> Add9/3
  Constant7/1 -> Product8/1
  Add8/1 -> Product8/2
  vx2/1 -> Add6/2, Add8/2, Add7/1
  Constant8/1 -> Product9/2
  Add7/1 -> Product9/1
  vx4/1 -> Add8/1
  vx1/1 -> Add7/2
  vx6/1 -> Add6/1
  Constant9/1 -> Product7/1
  Add6/1 -> Product7/2
  Product7/1 -> Add9/1
  Product3/1 -> Add5/1
  Add1/1 -> Product3/2
  Constant5/1 -> Product3/1
  xx6/1 -> Add1/1
  xx1/1 -> Add2/2
  xx4/1 -> Add4/1
  Add5/1 -> Product6/2
  Add2/1 -> Product5/1
  Product1/1 -> Add/2
  Constant1/1 -> Product1/1
  Constant/1 -> Product6/1
  Product6/1 -> Add/1
  Constant4/1 -> Product5/2
  xx2/1 -> Add2/1, Add4/2, Add1/2
  Add4/1 -> Product4/2
  Constant3/1 -> Product4/1
  Product5/1 -> Add5/3
  Product4/1 -> Add5/2
  Add9/1 -> Product1/2
  Gain/1 -> utx/1
  Add/1 -> Gain/1

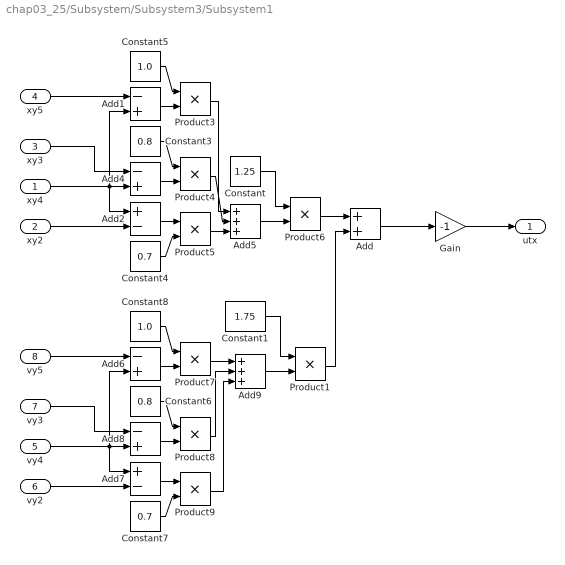
== system chap03_25/Subsystem/Subsystem3/Subsystem1 ==
  xy4 : Inport
  xy2 : Inport  Port=2
  xy3 : Inport  Port=3
  xy5 : Inport  Port=4
  vy4 : Inport  Port=5
  vy2 : Inport  Port=6
  vy3 : Inport  Port=7
  vy5 : Inport  Port=8
  Add : Sum
  Add{1,4,6,8} (4 alike) : Sum  Inputs=-+
  Add2 : Sum  Inputs=+-
  Add5 : Sum  Inputs=+++
  Add7 : Sum  Inputs=+-
  Add9 : Sum  Inputs=+++
  Constant : Constant  Value=1.25
  Constant1 : Constant  Value=1.75
  Constant3 : Constant  Value=0.8
  Constant4 : Constant  Value=0.7
  Constant5 : Constant  Value=1.0
  Constant6 : Constant  Value=0.8
  Constant7 : Constant  Value=0.7
  Constant8 : Constant  Value=1.0
  Gain : Gain  Gain=-1
  Product{1,3..9} (8 alike) : Product
  utx : Outport
  wires:
  Add9/1 -> Product1/2
  Product4/1 -> Add5/2
  Product5/1 -> Add5/3
  Constant3/1 -> Product4/1
  Add4/1 -> Product4/2
  xy4/1 -> Add1/2, Add4/2, Add2/1
  Constant4/1 -> Product5/2
  Product6/1 -> Add/1
  Constant/1 -> Product6/1
  Constant1/1 -> Product1/1
  Product1/1 -> Add/2
  Add2/1 -> Product5/1
  Add5/1 -> Product6/2
  xy3/1 -> Add4/1
  xy2/1 -> Add2/2
  xy5/1 -> Add1/1
  Constant5/1 -> Product3/1
  Add1/1 -> Product3/2
  Product3/1 -> Add5/1
  Product7/1 -> Add9/1
  Add6/1 -> Product7/2
  Constant8/1 -> Product7/1
  vy5/1 -> Add6/1
  vy2/1 -> Add7/2
  vy3/1 -> Add8/1
  Add7/1 -> Product9/1
  Constant7/1 -> Product9/2
  vy4/1 -> Add7/1, Add8/2, Add6/2
  Add8/1 -> Product8/2
  Constant6/1 -> Product8/1
  Product9/1 -> Add9/3
  Product8/1 -> Add9/2
  Gain/1 -> utx/1
  Add/1 -> Gain/1

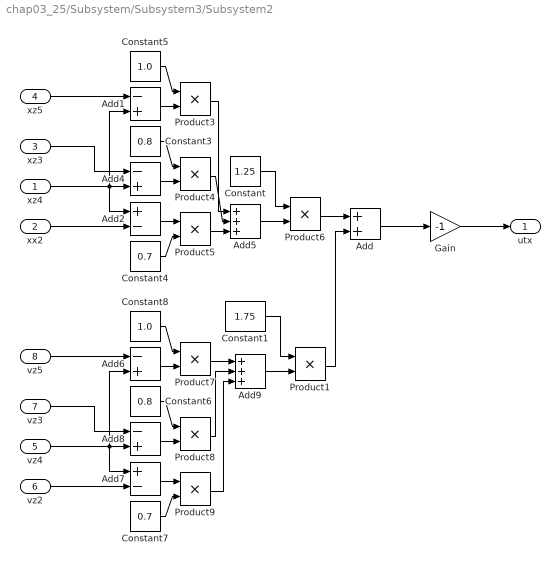
== system chap03_25/Subsystem/Subsystem3/Subsystem2 ==
  xz4 : Inport
  xx2 : Inport  Port=2
  xz3 : Inport  Port=3
  xz5 : Inport  Port=4
  vz4 : Inport  Port=5
  vz2 : Inport  Port=6
  vz3 : Inport  Port=7
  vz5 : Inport  Port=8
  Add : Sum
  Add{1,4,6,8} (4 alike) : Sum  Inputs=-+
  Add2 : Sum  Inputs=+-
  Add5 : Sum  Inputs=+++
  Add7 : Sum  Inputs=+-
  Add9 : Sum  Inputs=+++
  Constant : Constant  Value=1.25
  Constant1 : Constant  Value=1.75
  Constant3 : Constant  Value=0.8
  Constant4 : Constant  Value=0.7
  Constant5 : Constant  Value=1.0
  Constant6 : Constant  Value=0.8
  Constant7 : Constant  Value=0.7
  Constant8 : Constant  Value=1.0
  Gain : Gain  Gain=-1
  Product{1,3..9} (8 alike) : Product
  utx : Outport
  wires:
  Product8/1 -> Add9/2
  Product9/1 -> Add9/3
  Constant6/1 -> Product8/1
  Add8/1 -> Product8/2
  vz4/1 -> Add6/2, Add8/2, Add7/1
  Constant7/1 -> Product9/2
  Add7/1 -> Product9/1
  vz3/1 -> Add8/1
  vz2/1 -> Add7/2
  vz5/1 -> Add6/1
  Constant8/1 -> Product7/1
  Add6/1 -> Product7/2
  Product7/1 -> Add9/1
  Product3/1 -> Add5/1
  Add1/1 -> Product3/2
  Constant5/1 -> Product3/1
  xz5/1 -> Add1/1
  xx2/1 -> Add2/2
  xz3/1 -> Add4/1
  Add5/1 -> Product6/2
  Add2/1 -> Product5/1
  Product1/1 -> Add/2
  Constant1/1 -> Product1/1
  Constant/1 -> Product6/1
  Product6/1 -> Add/1
  Constant4/1 -> Product5/2
  xz4/1 -> Add2/1, Add4/2, Add1/2
  Add4/1 -> Product4/2
  Constant3/1 -> Product4/1
  Product5/1 -> Add5/3
  Product4/1 -> Add5/2
  Add9/1 -> Product1/2
  Gain/1 -> utx/1
  Add/1 -> Gain/1

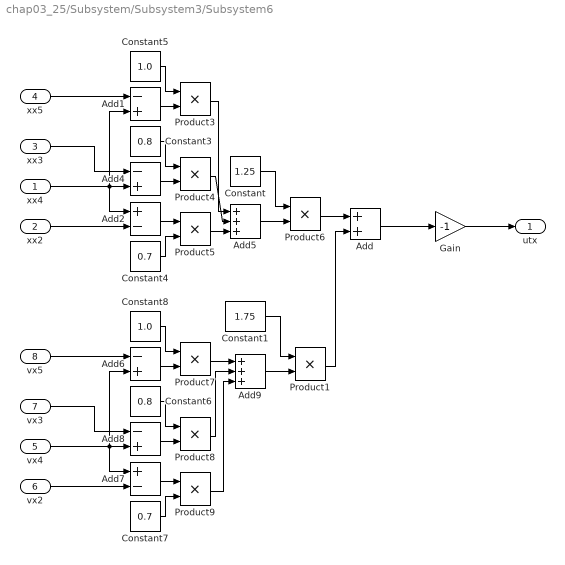
== system chap03_25/Subsystem/Subsystem3/Subsystem6 ==
  xx4 : Inport
  xx2 : Inport  Port=2
  xx3 : Inport  Port=3
  xx5 : Inport  Port=4
  vx4 : Inport  Port=5
  vx2 : Inport  Port=6
  vx3 : Inport  Port=7
  vx5 : Inport  Port=8
  Add : Sum
  Add{1,4,6,8} (4 alike) : Sum  Inputs=-+
  Add2 : Sum  Inputs=+-
  Add5 : Sum  Inputs=+++
  Add7 : Sum  Inputs=+-
  Add9 : Sum  Inputs=+++
  Constant : Constant  Value=1.25
  Constant1 : Constant  Value=1.75
  Constant3 : Constant  Value=0.8
  Constant4 : Constant  Value=0.7
  Constant5 : Constant  Value=1.0
  Constant6 : Constant  Value=0.8
  Constant7 : Constant  Value=0.7
  Constant8 : Constant  Value=1.0
  Gain : Gain  Gain=-1
  Product{1,3..9} (8 alike) : Product
  utx : Outport
  wires:
  Product8/1 -> Add9/2
  Product9/1 -> Add9/3
  Constant6/1 -> Product8/1
  Add8/1 -> Product8/2
  vx4/1 -> Add6/2, Add8/2, Add7/1
  Constant7/1 -> Product9/2
  Add7/1 -> Product9/1
  vx3/1 -> Add8/1
  vx2/1 -> Add7/2
  vx5/1 -> Add6/1
  Constant8/1 -> Product7/1
  Add6/1 -> Product7/2
  Product7/1 -> Add9/1
  Product3/1 -> Add5/1
  Add1/1 -> Product3/2
  Constant5/1 -> Product3/1
  xx5/1 -> Add1/1
  xx2/1 -> Add2/2
  xx3/1 -> Add4/1
  Add5/1 -> Product6/2
  Add2/1 -> Product5/1
  Product1/1 -> Add/2
  Constant1/1 -> Product1/1
  Constant/1 -> Product6/1
  Product6/1 -> Add/1
  Constant4/1 -> Product5/2
  xx4/1 -> Add2/1, Add4/2, Add1/2
  Add4/1 -> Product4/2
  Constant3/1 -> Product4/1
  Product5/1 -> Add5/3
  Product4/1 -> Add5/2
  Add9/1 -> Product1/2
  Gain/1 -> utx/1
  Add/1 -> Gain/1

== system chap03_25/Subsystem/Subsystem4/Subsystem1 ==
  xy6 : Inport
  xy1 : Inport  Port=2
  xy2 : Inport  Port=3
  vy6 : Inport  Port=4
  vy1 : Inport  Port=5
  vy2 : Inport  Port=6
  Add : Sum
  Add10 : Sum  Inputs=-+
  Add2 : Sum  Inputs=+-
  Add4 : Sum  Inputs=-+
  Add5 : Sum
  Add8 : Sum
  Add9 : Sum  Inputs=+-
  Constant : Constant  Value=1.25
  Constant1 : Constant  Value=1.75
  Constant3 : Constant  Value=1.0
  Constant4 : Constant  Value=1.2
  Constant5 : Constant  Value=1.2
  Constant6 : Constant  Value=1.0
  Gain : Gain  Gain=-1
  Product{1,4..6,8..9} (6 alike) : Product
  uty : Outport
  wires:
  vy6/1 -> Add9/1, Add10/2
  vy2/1 -> Add10/1
  vy1/1 -> Add9/2
  xy1/1 -> Add2/2
  xy2/1 -> Add4/1
  Add5/1 -> Product6/2
  Add2/1 -> Product5/1
  Product1/1 -> Add/2
  Constant1/1 -> Product1/1
  Constant/1 -> Product6/1
  Product6/1 -> Add/1
  Constant3/1 -> Product5/2
  xy6/1 -> Add4/2, Add2/1
  Add4/1 -> Product4/2
  Constant4/1 -> Product4/1
  Product5/1 -> Add5/2
  Product4/1 -> Add5/1
  Add8/1 -> Product1/2
  Constant5/1 -> Product8/1
  Add10/1 -> Product8/2
  Constant6/1 -> Product9/2
  Add9/1 -> Product9/1
  Product8/1 -> Add8/1
  Product9/1 -> Add8/2
  Gain/1 -> uty/1
  Add/1 -> Gain/1

== system chap03_25/Subsystem/Subsystem4/Subsystem2 ==
  xz6 : Inport
  xz1 : Inport  Port=2
  xz2 : Inport  Port=3
  vz6 : Inport  Port=4
  vz1 : Inport  Port=5
  vz2 : Inport  Port=6
  Add : Sum
  Add10 : Sum  Inputs=-+
  Add2 : Sum  Inputs=+-
  Add4 : Sum  Inputs=-+
  Add5 : Sum
  Add8 : Sum
  Add9 : Sum  Inputs=+-
  Constant : Constant  Value=1.25
  Constant1 : Constant  Value=1.75
  Constant3 : Constant  Value=1.0
  Constant4 : Constant  Value=1.2
  Constant5 : Constant  Value=1.2
  Constant6 : Constant  Value=1.0
  Gain : Gain  Gain=-1
  Product{1,4..6,8..9} (6 alike) : Product
  utz : Outport
  wires:
  Product9/1 -> Add8/2
  Product8/1 -> Add8/1
  Add9/1 -> Product9/1
  Constant6/1 -> Product9/2
  Add10/1 -> Product8/2
  Constant5/1 -> Product8/1
  Add8/1 -> Product1/2
  Product4/1 -> Add5/1
  Product5/1 -> Add5/2
  Constant4/1 -> Product4/1
  Add4/1 -> Product4/2
  xz6/1 -> Add2/1, Add4/2
  Constant3/1 -> Product5/2
  Product6/1 -> Add/1
  Constant/1 -> Product6/1
  Constant1/1 -> Product1/1
  Product1/1 -> Add/2
  Add2/1 -> Product5/1
  Add5/1 -> Product6/2
  xz2/1 -> Add4/1
  xz1/1 -> Add2/2
  vz1/1 -> Add9/2
  vz2/1 -> Add10/1
  vz6/1 -> Add10/2, Add9/1
  Gain/1 -> utz/1
  Add/1 -> Gain/1

== system chap03_25/Subsystem/Subsystem4/Subsystem6 ==
  xx6 : Inport
  xx1 : Inport  Port=2
  xx2 : Inport  Port=3
  vx6 : Inport  Port=4
  vx1 : Inport  Port=5
  vx2 : Inport  Port=6
  Add : Sum
  Add10 : Sum  Inputs=-+
  Add2 : Sum  Inputs=+-
  Add4 : Sum  Inputs=-+
  Add5 : Sum
  Add8 : Sum
  Add9 : Sum  Inputs=+-
  Constant : Constant  Value=1.25
  Constant1 : Constant  Value=1.75
  Constant3 : Constant  Value=1.0
  Constant4 : Constant  Value=1.2
  Constant5 : Constant  Value=1.2
  Constant6 : Constant  Value=1.0
  Gain : Gain  Gain=-1
  Product{1,4..6,8..9} (6 alike) : Product
  utx : Outport
  wires:
  Product9/1 -> Add8/2
  Product8/1 -> Add8/1
  Add9/1 -> Product9/1
  Constant6/1 -> Product9/2
  Add10/1 -> Product8/2
  Constant5/1 -> Product8/1
  Add8/1 -> Product1/2
  Product4/1 -> Add5/1
  Product5/1 -> Add5/2
  Constant4/1 -> Product4/1
  Add4/1 -> Product4/2
  xx6/1 -> Add2/1, Add4/2
  Constant3/1 -> Product5/2
  Product6/1 -> Add/1
  Constant/1 -> Product6/1
  Constant1/1 -> Product1/1
  Product1/1 -> Add/2
  Add2/1 -> Product5/1
  Add5/1 -> Product6/2
  xx2/1 -> Add4/1
  xx1/1 -> Add2/2
  vx1/1 -> Add9/2
  vx2/1 -> Add10/1
  vx6/1 -> Add10/2, Add9/1
  Gain/1 -> utx/1
  Add/1 -> Gain/1

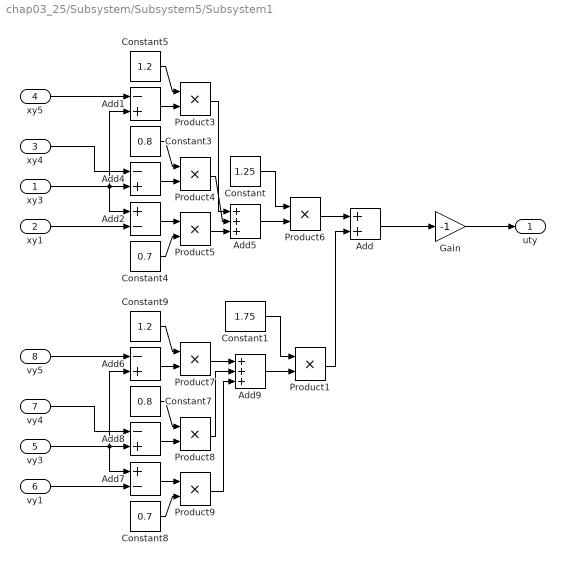
== system chap03_25/Subsystem/Subsystem5/Subsystem1 ==
  xy3 : Inport
  xy1 : Inport  Port=2
  xy4 : Inport  Port=3
  xy5 : Inport  Port=4
  vy3 : Inport  Port=5
  vy1 : Inport  Port=6
  vy4 : Inport  Port=7
  vy5 : Inport  Port=8
  Add : Sum
  Add{1,4,6,8} (4 alike) : Sum  Inputs=-+
  Add2 : Sum  Inputs=+-
  Add5 : Sum  Inputs=+++
  Add7 : Sum  Inputs=+-
  Add9 : Sum  Inputs=+++
  Constant : Constant  Value=1.25
  Constant1 : Constant  Value=1.75
  Constant3 : Constant  Value=0.8
  Constant4 : Constant  Value=0.7
  Constant5 : Constant  Value=1.2
  Constant7 : Constant  Value=0.8
  Constant8 : Constant  Value=0.7
  Constant9 : Constant  Value=1.2
  Gain : Gain  Gain=-1
  Product{1,3..9} (8 alike) : Product
  uty : Outport
  wires:
  Product8/1 -> Add9/2
  Product9/1 -> Add9/3
  Constant7/1 -> Product8/1
  Add8/1 -> Product8/2
  vy3/1 -> Add6/2, Add8/2, Add7/1
  Constant8/1 -> Product9/2
  Add7/1 -> Product9/1
  vy4/1 -> Add8/1
  vy1/1 -> Add7/2
  vy5/1 -> Add6/1
  Constant9/1 -> Product7/1
  Add6/1 -> Product7/2
  Product7/1 -> Add9/1
  Product3/1 -> Add5/1
  Add1/1 -> Product3/2
  Constant5/1 -> Product3/1
  xy5/1 -> Add1/1
  xy1/1 -> Add2/2
  xy4/1 -> Add4/1
  Add5/1 -> Product6/2
  Add2/1 -> Product5/1
  Product1/1 -> Add/2
  Constant1/1 -> Product1/1
  Constant/1 -> Product6/1
  Product6/1 -> Add/1
  Constant4/1 -> Product5/2
  xy3/1 -> Add2/1, Add4/2, Add1/2
  Add4/1 -> Product4/2
  Constant3/1 -> Product4/1
  Product5/1 -> Add5/3
  Product4/1 -> Add5/2
  Add9/1 -> Product1/2
  Gain/1 -> uty/1
  Add/1 -> Gain/1
